simulink model "simulation"  (R2023a)
settings: Solver=ode45  StartTime=0.0  StopTime=1  MaxStep=0.2  RelTol=1e-3
settings Model: Creator=glebari  LastModifiedBy=glebari

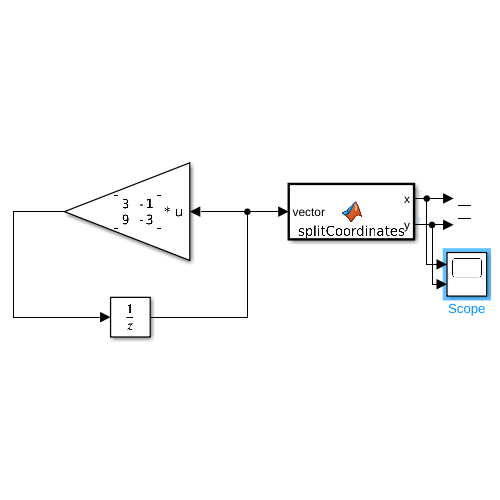
[thumbnail: Simulink's stored preview of the top-level diagram]
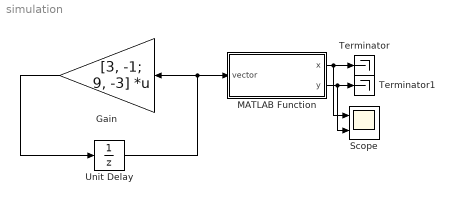
== system simulation ==
  Gain : Gain  Gain=[3, -1; 9, -3]  Multiplication=Matrix(K*u)
  MATLAB Function : MATLAB Function  TreatAsAtomicUnit=on
  Scope : Scope  NumInputPorts=2
  Terminator : Terminator
  Terminator1 : Terminator
  Unit Delay : UnitDelay  InitialCondition=[-0.5; 3]  SampleTime=-1  HasFrameUpgradeWarning=on
  wires:
  Gain/1 -> Unit Delay/1
  Unit Delay/1 -> MATLAB Function/1(vector), Gain/1
  MATLAB Function/1(x) -> Scope/1, Terminator/1
  MATLAB Function/2(y) -> Scope/2, Terminator1/1

== matlab function simulation/MATLAB Function ==
  data: x output; vector input; y output
function [x, y] = splitCoordinates(vector)
    x = vector(1);
    y = vector(2);
end
